simulink model "matlab_function_in_simulink"  (R2021a)
settings: Solver=VariableStepAuto  StartTime=0.0  StopTime=10.0  RelTol=1e-3
settings Model: Creator=jun  LastModifiedBy=jun

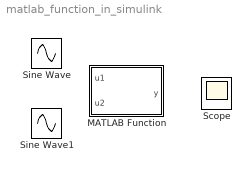
== system matlab_function_in_simulink ==
  MATLAB Function : MATLAB Function  TreatAsAtomicUnit=on
  Scope : Scope
  Sine Wave : Sin  SampleTime=0
  Sine Wave1 : Sin  SampleTime=0

== matlab function matlab_function_in_simulink/MATLAB Function ==
  data: u1 input; y output; u2 input
function y = fcn(u1, u2)
%#codegen

y = u1 + u2;
